simulink model "SIR_on_off"  (R2018b)
settings: Solver=ode4  StartTime=0.0  StopTime=200  FixedStep=0.1  RelTol=1e-3
settings Model: Creator=emcoates  LastModifiedBy=emcoates

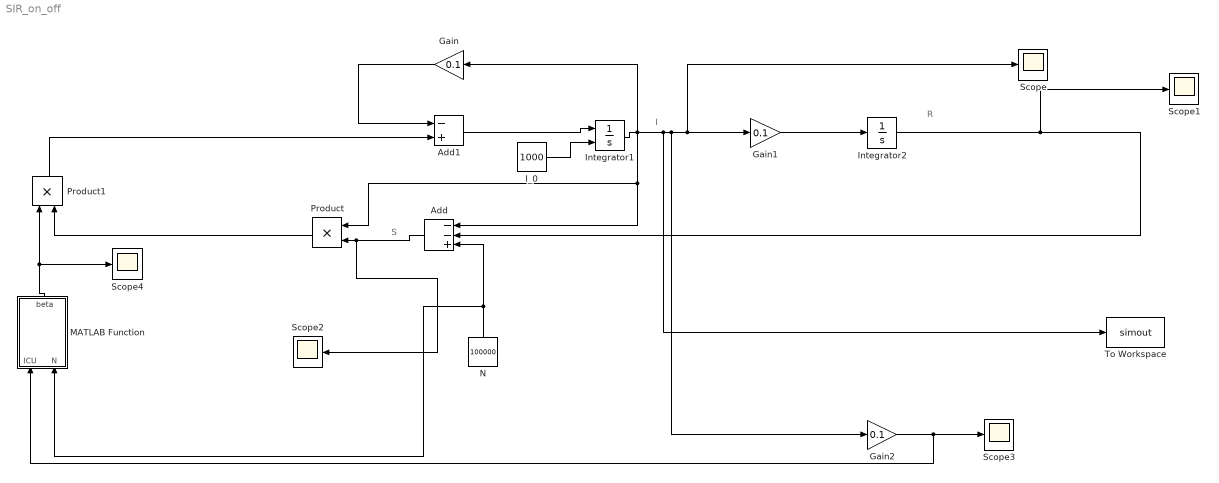
== system SIR_on_off ==
  note: R
  note: I
  note: S
  Add : Sum  Inputs=--+
  Add1 : Sum  Inputs=-+
  Gain : Gain  Gain=0.1
  Gain1 : Gain  Gain=0.1
  Gain2 : Gain  Gain=0.1
  I_0 : Constant  Value=1000
  Integrator1 : Integrator  InitialConditionSource=external
  Integrator2 : Integrator
  MATLAB Function : MATLAB Function  TreatAsAtomicUnit=on
  N : Constant  Value=100000
  Product : Product
  Product1 : Product
  Scope{,1..4} (5 alike) : Scope
  To Workspace : ToWorkspace  VariableName=simout  SaveFormat=Timeseries  SampleTime=-1
  wires:
  N/1 -> MATLAB Function/2(N), Add/3
  Integrator2/1 -> Scope1/1, Add/2
  Integrator1/1 -> To Workspace/1, Gain2/1, Scope/1, Gain1/1, Product/1, Add/1, Gain/1
  Add/1 -> Scope2/1, Product/2
  Gain/1 -> Add1/1
  Add1/1 -> Integrator1/1
  Gain1/1 -> Integrator2/1
  I_0/1 -> Integrator1/2
  Gain2/1 -> MATLAB Function/1(ICU), Scope3/1
  MATLAB Function/1(beta) -> Scope4/1, Product1/1
  Product/1 -> Product1/2
  Product1/1 -> Add1/2

== matlab function SIR_on_off/MATLAB Function ==
  settings: updateMethod=DISCRETE
  data: ICU input; beta output; N input
function beta = fcn(ICU,N)

persistent state;

if(isempty(state))
    state = 0;
end

u = 0;
if(ICU<5)
    % slipp opp
    u = 0;
    state = 1; % going up 
elseif(ICU < 20) % but not less than 5
    if(~state) % going down
        u = 1;
    else % state == 1 going up
        u = 0;
    end
else % >= 6
    % stram inn
    u = 1;
    state = 0; % going down
end
    
beta_2 = 0.01/N;
beta_1 = 0.23/N;

beta = beta_2*u + beta_1*(1-u);
end
